simulink model "c_lab8sim"  (R2020b)
settings: Solver=FixedStepAuto  StartTime=0.0  StopTime=100  FixedStep=0.0001  RelTol=1e-3
libraries: simulink x1
settings Model: Creator=musa oğural  LastModifiedBy=musa oğural

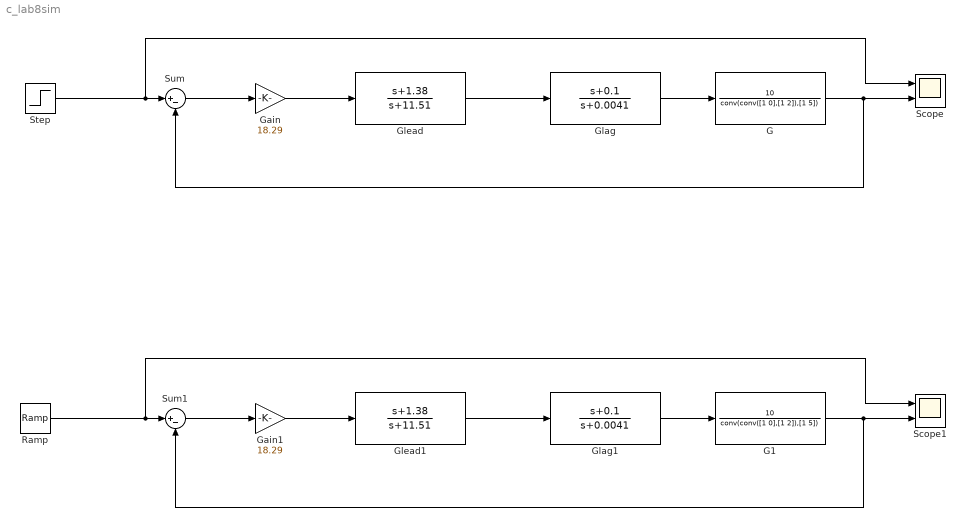
== system c_lab8sim ==
  G : TransferFcn  Numerator=[10]  Denominator=conv(conv([1 0],[1 2]),[1 5])
  G1 : TransferFcn  Numerator=[10]  Denominator=conv(conv([1 0],[1 2]),[1 5])
  Gain : Gain  Gain=18.29
  Gain1 : Gain  Gain=18.29
  Glag : TransferFcn  Numerator=[1 0.1]  Denominator=[1 0.0041]
  Glag1 : TransferFcn  Numerator=[1 0.1]  Denominator=[1 0.0041]
  Glead : TransferFcn  Numerator=[1 1.38]  Denominator=[1 11.51]
  Glead1 : TransferFcn  Numerator=[1 1.38]  Denominator=[1 11.51]
  Ramp : simulink/Sources/Ramp  slope=1  start=0  InitialOutput=0
  Scope : Scope  NumInputPorts=2
  Scope1 : Scope  NumInputPorts=2
  Step : Step  Time=0  SampleTime=0
  Sum : Sum  Inputs=|+-
  Sum1 : Sum  Inputs=|+-
  wires:
  Sum/1 -> Gain/1
  Gain/1 -> Glead/1
  Glead/1 -> Glag/1
  Glag/1 -> G/1
  G/1 -> Sum/2, Scope/2
  Step/1 -> Scope/1, Sum/1
  Glag1/1 -> G1/1
  Glead1/1 -> Glag1/1
  Sum1/1 -> Gain1/1
  Gain1/1 -> Glead1/1
  G1/1 -> Sum1/2, Scope1/2
  Ramp/1 -> Scope1/1, Sum1/1
